simulink model "simulator"  (Simulink 8.4)
settings: Solver=ode45  StartTime=0.0  StopTime=20  FixedStep=0.05  RelTol=1e-3
values from neighbouring files (symbols this model uses):
  A = [A;T*Rkc]    [CG.m]    (also in CGOffLineSetting.m = [eye(length(dmax));-eye(length(dmax))]; makeSystem.m = [0 1 0 0)
  B = [dmax;-dmax]    [CGOffLineSetting.m]    (also in makeSystem.m = [0;0;0;kt/(R*JM)])
  delta = 0.000001    (= 1e-06)    [main.m]    (also in makeSystem.m = 1e-08)
  dimCon = length(g)/2    [makeSystem.m]
  dimRef = 1    [makeSystem.m]
  dimSys = length(Phi)    [makeSystem.m]
  g = p    [CG.m]    (also in CGYalmip.m = double(W); makeSystem.m = [78.5398;220;78.5398;220])
  G = sys2.b    [makeSystem.m]
  Hc = [Hy(2:3,:)]    [makeSystem.m]
  Hy = C    [makeSystem.m]
  k0 = k    (= 1)    [CGOffLineSetting.m]    (also in main.m = 10)
  L = [D(2:3,1)]    [makeSystem.m]
  Phi = sys2.a    [makeSystem.m]
  Psi = 1    [makeSystem.m]
  reference = pi/2    (= 1.57079632679)    [makeSystem.m]
  T = [1 0; 0 1;-1 0;0 -1]    [makeSystem.m]
  Ts = 0.1    [makeSystem.m]
undefined symbols (not defined in the file or in its folder): Ac, Bc, Cc, CGYalmip
settings Model: Creator=francesco  LastModifiedBy=Gianni  ExtModeAutoUpdateStatusClock=off
settings DebuggingCC: SaveWithParameterizedLinksMsg=none

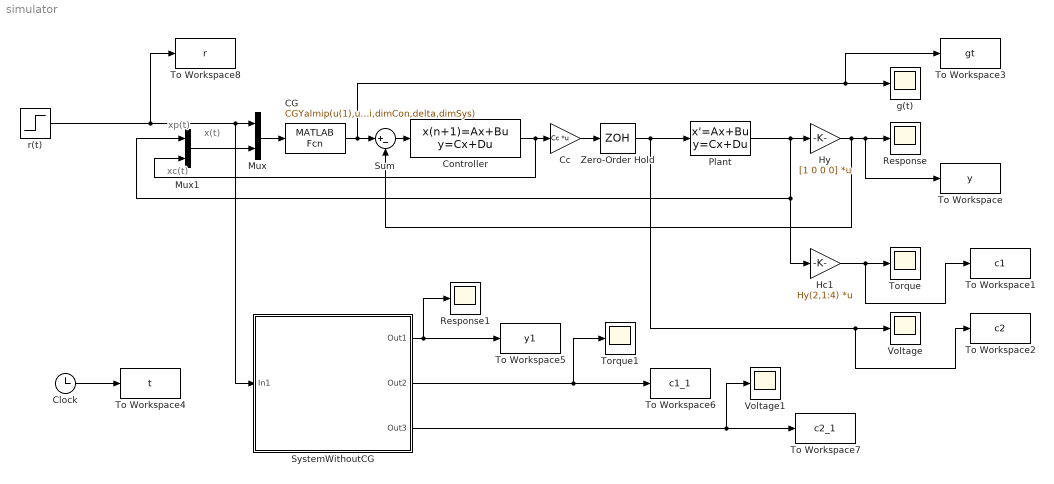
== system simulator ==
  note: xc(t)
  note: xp(t)
  note: x(t)
  CG : MATLABFcn  MATLABFcn=CGYalmip(u(1),u(2:9),g,T,Hc,Phi,G,L,k0,dimRef,Psi,dimCon,delta,dimSys)  OutputDimensions=1  SampleTime=Ts
  Cc : Gain  Gain=Cc  Multiplication=Matrix(K*u) (u vector)  SampleTime=Ts
  Clock : Clock
  Controller : DiscreteStateSpace  A=Ac  B=Bc  C=eye(4)  D=[0;0;0;0]  SampleTime=Ts
  Hc1 : Gain  Gain=Hy(2,1:4)  Multiplication=Matrix(K*u) (u vector)
  Hy : Gain  Gain=[1 0 0 0]  Multiplication=Matrix(K*u) (u vector)
  Mux : Mux  Inputs=2
  Mux1 : Mux  Inputs=2
  Plant : StateSpace  A=A  B=B  C=eye(4)  D=[0 0 0 0]'  X0=0
  Response : Scope
      settings: YMin=1.425  YMax=1.825
  Response1 : Scope
  Sum : Sum  Inputs=|+-
  SystemWithoutCG : Subsystem
  To Workspace : ToWorkspace  VariableName=y  SampleTime=-1
  To Workspace1 : ToWorkspace  VariableName=c1  SampleTime=-1
  To Workspace2 : ToWorkspace  VariableName=c2  SampleTime=-1
  To Workspace3 : ToWorkspace  VariableName=gt  SampleTime=-1
  To Workspace4 : ToWorkspace  VariableName=t  SampleTime=-1
  To Workspace5 : ToWorkspace  VariableName=y1  SampleTime=-1
  To Workspace6 : ToWorkspace  VariableName=c1_1  SampleTime=-1
  To Workspace7 : ToWorkspace  VariableName=c2_1  SampleTime=-1
  To Workspace8 : ToWorkspace  VariableName=r  SampleTime=-1
  Torque : Scope
      settings: TimeRange=6  YMin=-0.12  YMax=-0.045  SaveName=ScopeData2
  Torque1 : Scope
      settings: SaveName=ScopeData5
  Voltage : Scope
      settings: SaveName=ScopeData4
  Voltage1 : Scope
      settings: SaveName=ScopeData6
  Zero-Order Hold : ZeroOrderHold  SampleTime=Ts
  g(t) : Scope
      settings: YMin=1.49226  YMax=1.64934  SaveName=ScopeData3
  r(t) : Step  Time=0  After=reference  SampleTime=Ts
  wires:
  Plant/1 -> Hy/1, Hc1/1, Mux1/1
  r(t)/1 -> To Workspace8/1, Mux/1, SystemWithoutCG/1(In1)
  Mux1/1 -> Mux/2
  Controller/1 -> Mux1/2, Cc/1
  Mux/1 -> CG/1
  CG/1 -> g(t)/1, To Workspace3/1, Sum/1
  Hy/1 -> Sum/2, Response/1, To Workspace/1
  Hc1/1 -> Torque/1, To Workspace1/1
  Cc/1 -> Zero-Order Hold/1
  Zero-Order Hold/1 -> Voltage/1, To Workspace2/1, Plant/1
  Clock/1 -> To Workspace4/1
  SystemWithoutCG/2(Out2) -> To Workspace6/1, Torque1/1
  SystemWithoutCG/1(Out1) -> To Workspace5/1, Response1/1
  SystemWithoutCG/3(Out3) -> To Workspace7/1, Voltage1/1
  Sum/1 -> Controller/1

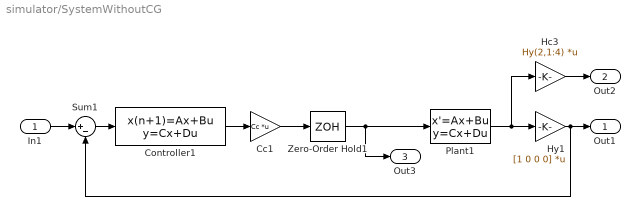
== system simulator/SystemWithoutCG ==
  In1 : Inport
  Cc1 : Gain  Gain=Cc  Multiplication=Matrix(K*u) (u vector)  SampleTime=Ts
  Controller1 : DiscreteStateSpace  A=Ac  B=Bc  C=eye(4)  D=[0;0;0;0]  SampleTime=Ts
  Hc3 : Gain  Gain=Hy(2,1:4)  Multiplication=Matrix(K*u) (u vector)
  Hy1 : Gain  Gain=[1 0 0 0]  Multiplication=Matrix(K*u) (u vector)
  Plant1 : StateSpace  A=A  B=B  C=eye(4)  D=[0 0 0 0]'  X0=0
  Sum1 : Sum  Inputs=|+-
  Zero-Order Hold1 : ZeroOrderHold  SampleTime=Ts
  Out1 : Outport
  Out2 : Outport  Port=2
  Out3 : Outport  Port=3
  wires:
  Plant1/1 -> Hy1/1, Hc3/1
  Sum1/1 -> Controller1/1
  Controller1/1 -> Cc1/1
  Hy1/1 -> Sum1/2, Out1/1
  Cc1/1 -> Zero-Order Hold1/1
  Zero-Order Hold1/1 -> Out3/1, Plant1/1
  In1/1 -> Sum1/1
  Hc3/1 -> Out2/1
